simulink model "HFV_Injection_2015a"  (R2016a)
settings: Solver=ode3  SolverMode=SingleTasking  StartTime=0.0  StopTime=5  FixedStep=Simulation_Step  RelTol=1e-3
values from neighbouring files (symbols this model uses):
  Dm = 1e-4    (= 0.0001)    [param.m]
  HF = 400    [param.m]
  Jm = 2e-4    (= 0.0002)    [param.m]
  Ke = 0.002    [param.m]
  ki = wpll^2    (= 15791.3670417)    [param.m]
  kp = 2 * wpll    (= 251.327412287)    [param.m]
  Ld = 0.00019    [aaa.mat]    (also in param.m = 2e-05)
  Lq = 0.00051    [aaa.mat]    (also in param.m = 4e-05)
  omega = 100    [param.m]
  Pn = 4    [param.m]
  Qvalue = 1    [param.m]
  R = 2e-3    (= 0.002)    [param.m]
  tau = 1/Fc/2/pi    (= 0.00795774715459)    [param.m]
  tau_spd = 1/Fspd/2/pi    (= 0.0318309886184)    [param.m]
  Vh = 0.1    [param.m]
  w0 = HF * 2 * pi    (= 2513.27412287)    [param.m]
  wlpf = 20 * 2 * pi    (= 125.663706144)    [param.m]
settings Model: Creator=r720r  LastModifiedBy=Lenovo
settings DebuggingCC: SFUnexpectedBacktrackingDiag=error  SFNoUnconditionalDefaultTransitionDiag=error
settings HardwareCC: ProdWordSize=32  ProdHWDeviceType=Specified
settings SFSimCC: SimUseLocalCustomCode=on
settings RTWCC: RTWUseLocalCustomCode=on
settings GRTTargetCC: TargetLangStandard=C99 (ISO)  GeneratePreprocessorConditionals=Use local settings
settings ConfigComp: CovMetricSettings=dwe  CovHtmlReporting=off  CovSaveCumulativeToWorkspaceVar=off  CovSaveSingleToWorkspaceVar=off  CovModelRefEnable=Off  CovExternalEMLEnable=on

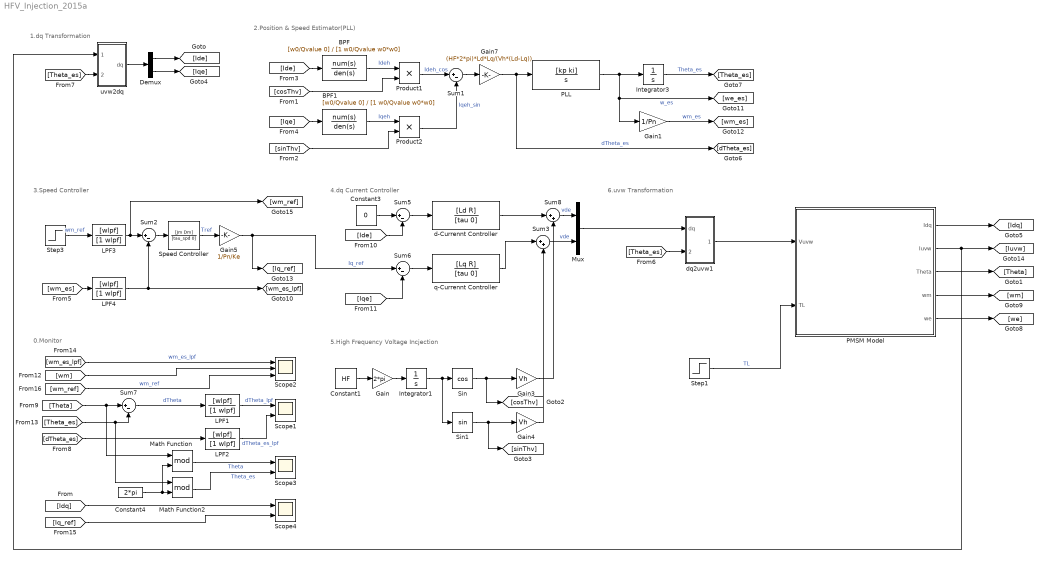
== system HFV_Injection_2015a ==
  note: 0.Monitor
  note: 6.uvw Transformation
  note: 1.dq Transformation
  note: 4.dq Current Controller
  note: 3.Speed Controller
  note: 5.High Frequency Voltage Incjection
  note: 2.Position & Speed Estimator(PLL)
  BPF : TransferFcn  Numerator=[w0/Qvalue 0]  Denominator=[1 w0/Qvalue w0*w0]
  BPF1 : TransferFcn  Numerator=[w0/Qvalue 0]  Denominator=[1 w0/Qvalue w0*w0]
  Constant1 : Constant  Value=HF
  Constant3 : Constant  Value=0
  Constant4 : Constant  Value=2*pi
  Demux : Demux  Outputs=2
  Gain : Gain  Gain=2*pi
  Gain1 : Gain  Gain=1/Pn
  Gain3 : Gain  Gain=Vh
  Gain4 : Gain  Gain=Vh
  Gain5 : Gain  Gain=1/Pn/Ke
  Gain7 : Gain  Gain=(HF*2*pi)*Ld*Lq/(Vh*(Ld-Lq))
  Integrator1 : Integrator
  Integrator3 : Integrator
  LPF{1..4} (4 alike) : TransferFcn  Numerator=[wlpf]  Denominator=[1 wlpf]
  Math Function : Math  Operator=mod  SaturateOnIntegerOverflow=on
  Math Function2 : Math  Operator=mod  SaturateOnIntegerOverflow=on
  Mux : Mux  Inputs=2
  PLL : TransferFcn  Numerator=[kp ki]  Denominator=[1 0]
  PMSM Model : Subsystem
  Product1 : Product
  Product2 : Product
  Scope1 : Scope  NumInputPorts=2
  Scope2 : Scope  NumInputPorts=3
  Scope3 : Scope  NumInputPorts=2
  Scope4 : Scope  NumInputPorts=2
  Sin : Trigonometry  Operator=cos
  Sin1 : Trigonometry
  Speed Controller : TransferFcn  Numerator=[Jm Dm]  Denominator=[tau_spd 0]
  Step1 : Step  Time=3  After=0.01  SampleTime=0
  Step3 : Step  Time=0.2  After=omega/Pn  SampleTime=0
  Sum{1..2,5..7} (5 alike) : Sum  Inputs=|+-
  Sum3 : Sum  Inputs=|++
  Sum8 : Sum  Inputs=|++
  d-Currennt Controller : TransferFcn  Numerator=[Ld R]  Denominator=[tau 0]
  dq2uvw1 : Subsystem
  q-Currennt Controller : TransferFcn  Numerator=[Lq R]  Denominator=[tau 0]
  uvw2dq : Subsystem
  wires:
  Sin/1 -> [cosThv], Gain3/1
  Sin1/1 -> [sinThv], Gain4/1
  Integrator1/1 -> Sin1/1, Sin/1
  Gain/1 -> Integrator1/1
  Constant1/1 -> Gain/1
  [cosThv] -> Product1/2
  BPF/1 -> Product1/1  "Ideh"
  BPF1/1 -> Product2/1  "Iqeh"
  [sinThv] -> Product2/2
  Product1/1 -> Sum1/1  "Ideh_cos"
  Product2/1 -> Sum1/2  "Iqeh_sin"
  Sum1/1 -> Gain7/1
  Gain7/1 -> [dTheta_es], PLL/1  "dTheta_es"
  PLL/1 -> Gain1/1, [we_es], Integrator3/1  "w_es"
  Integrator3/1 -> [Theta_es]  "Theta_es"
  [Ide] -> BPF/1
  [Iqe] -> BPF1/1
  [Theta_es] -> dq2uvw1/2(Theta)
  dq2uvw1/1(uvw) -> PMSM Model/1(Vuvw)
  Sum8/1 -> Mux/1  "vde"
  d-Currennt Controller/1 -> Sum8/1
  Sum3/1 -> Mux/2  "vde"
  q-Currennt Controller/1 -> Sum3/1
  Constant3/1 -> Sum5/1
  Sum5/1 -> d-Currennt Controller/1
  [Ide] -> Sum5/2
  Sum6/1 -> q-Currennt Controller/1
  [Iqe] -> Sum6/2
  [Theta] -> Math Function/1, Sum7/1
  [Theta_es] -> Math Function2/1, Sum7/2
  Gain3/1 -> Sum8/2
  Gain4/1 -> Sum3/2
  Sum7/1 -> LPF1/1  "dTheta"
  LPF1/1 -> Scope1/1  "dTheta_lpf"
  LPF2/1 -> Scope1/2  "dTheta_es_lpf"
  PMSM Model/3(Theta) -> [Theta]
  PMSM Model/5(we) -> [we]
  PMSM Model/4(wm) -> [wm]
  Sum2/1 -> Speed Controller/1
  Gain1/1 -> [wm_es]  "wm_es"
  Speed Controller/1 -> Gain5/1  "Tref"
  Gain5/1 -> Sum6/1, [Iq_ref]  "Iq_ref"
  [wm] -> Scope2/2
  [wm_es] -> LPF4/1
  LPF4/1 -> [wm_es_lpf], Sum2/2
  PMSM Model/2(Iuvw) -> uvw2dq/1(uvw), [Iuvw]
  Mux/1 -> dq2uvw1/1(dq)
  uvw2dq/1(dq) -> Demux/1
  Demux/1 -> [Ide]
  Demux/2 -> [Iqe]
  [Theta_es] -> uvw2dq/2(Theta)
  PMSM Model/1(Idq) -> [Idq]
  [dTheta_es] -> LPF2/1
  Step3/1 -> LPF3/1  "wm_ref"
  LPF3/1 -> [wm_ref], Sum2/1
  Step1/1 -> PMSM Model/2(TL)  "TL"
  Constant4/1 -> Math Function2/2, Math Function/2
  Math Function/1 -> Scope3/1  "Theta"
  Math Function2/1 -> Scope3/2  "Theta_es"
  [Idq] -> Scope4/1
  [Iq_ref] -> Scope4/2
  [wm_es_lpf] -> Scope2/1  "wm_es_lpf"
  [wm_ref] -> Scope2/3  "wm_ref"

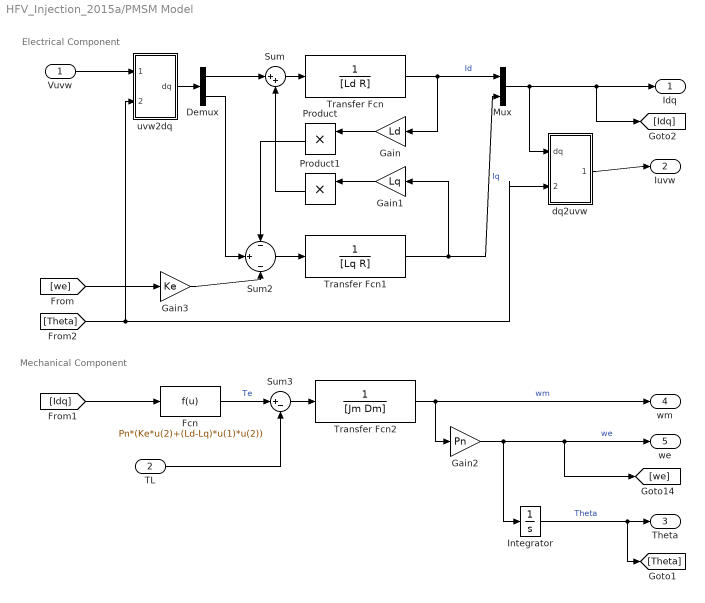
== system HFV_Injection_2015a/PMSM Model ==
  note: Mechanical Component
  note: Electrical Component
  Vuvw : Inport
  TL : Inport  Port=2
  Demux : Demux  Outputs=2
  Fcn : Fcn  Expr=Pn*(Ke*u(2)+(Ld-Lq)*u(1)*u(2))
  Gain : Gain  Gain=Ld
  Gain1 : Gain  Gain=Lq
  Gain2 : Gain  Gain=Pn
  Gain3 : Gain  Gain=Ke
  Integrator : Integrator
  Mux : Mux  Inputs=2
  Product : Product
  Product1 : Product
  Sum : Sum  Inputs=|++
  Sum2 : Sum  Inputs=-|+|-
  Sum3 : Sum  Inputs=|+-
  Transfer Fcn : TransferFcn  Denominator=[Ld R]
  Transfer Fcn1 : TransferFcn  Denominator=[Lq R]
  Transfer Fcn2 : TransferFcn  Denominator=[Jm Dm]
  dq2uvw : Subsystem
  uvw2dq : Subsystem
  Idq : Outport
  Iuvw : Outport  Port=2
  Theta : Outport  Port=3
  wm : Outport  Port=4
  we : Outport  Port=5
  wires:
  Product1/1 -> Sum/2
  Product/1 -> Sum2/1
  Transfer Fcn/1 -> Mux/1, Gain/1  "Id"
  Sum2/1 -> Transfer Fcn1/1
  Gain/1 -> Product/1
  Gain1/1 -> Product1/1
  Sum/1 -> Transfer Fcn/1
  Transfer Fcn1/1 -> Gain1/1, Mux/2  "Iq"
  Vuvw/1 -> uvw2dq/1(uvw)
  Mux/1 -> dq2uvw/1(dq), [Idq], Idq/1
  Fcn/1 -> Sum3/1  "Te"
  Transfer Fcn2/1 -> wm/1, Gain2/1  "wm"
  Gain2/1 -> Integrator/1, we/1, [we]  "we"
  Sum3/1 -> Transfer Fcn2/1
  TL/1 -> Sum3/2
  Gain3/1 -> Sum2/3
  Integrator/1 -> [Theta], Theta/1  "Theta"
  [we] -> Gain3/1
  [Idq] -> Fcn/1
  dq2uvw/1(uvw) -> Iuvw/1
  [Theta] -> dq2uvw/2(Theta), uvw2dq/2(Theta)
  uvw2dq/1(dq) -> Demux/1
  Demux/1 -> Sum/1
  Demux/2 -> Sum2/2

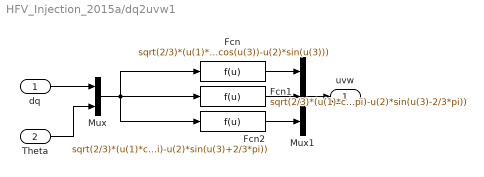
== system HFV_Injection_2015a/dq2uvw1 ==
  dq : Inport
  Theta : Inport  Port=2
  Fcn : Fcn  Expr=sqrt(2/3)*(u(1)*cos(u(3))-u(2)*sin(u(3)))
  Fcn1 : Fcn  Expr=sqrt(2/3)*(u(1)*cos(u(3)-2/3*pi)-u(2)*sin(u(3)-2/3*pi))
  Fcn2 : Fcn  Expr=sqrt(2/3)*(u(1)*cos(u(3)+2/3*pi)-u(2)*sin(u(3)+2/3*pi))
  Mux : Mux  Inputs=2
  Mux1 : Mux  Inputs=3
  uvw : Outport
  wires:
  dq/1 -> Mux/1
  Mux/1 -> Fcn2/1, Fcn/1, Fcn1/1
  Theta/1 -> Mux/2
  Fcn/1 -> Mux1/1
  Fcn1/1 -> Mux1/2
  Fcn2/1 -> Mux1/3
  Mux1/1 -> uvw/1

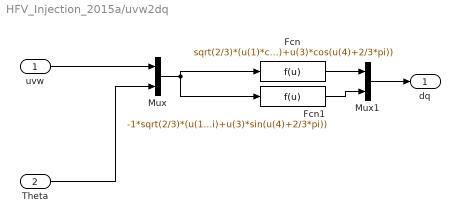
== system HFV_Injection_2015a/uvw2dq ==
  uvw : Inport
  Theta : Inport  Port=2
  Fcn : Fcn  Expr=sqrt(2/3)*(u(1)*cos(u(4))+u(2)*cos(u(4)-2/3*pi)+u(3)*cos(u(4)+2/3*pi))
  Fcn1 : Fcn  Expr=-1*sqrt(2/3)*(u(1)*sin(u(4))+u(2)*sin(u(4)-2/3*pi)+u(3)*sin(u(4)+2/3*pi))
  Mux : Mux  Inputs=2
  Mux1 : Mux  Inputs=2
  dq : Outport
  wires:
  uvw/1 -> Mux/1
  Mux/1 -> Fcn1/1, Fcn/1
  Fcn1/1 -> Mux1/2
  Fcn/1 -> Mux1/1
  Theta/1 -> Mux/2
  Mux1/1 -> dq/1

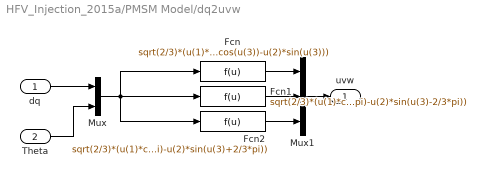
== system HFV_Injection_2015a/PMSM Model/dq2uvw ==
  dq : Inport
  Theta : Inport  Port=2
  Fcn : Fcn  Expr=sqrt(2/3)*(u(1)*cos(u(3))-u(2)*sin(u(3)))
  Fcn1 : Fcn  Expr=sqrt(2/3)*(u(1)*cos(u(3)-2/3*pi)-u(2)*sin(u(3)-2/3*pi))
  Fcn2 : Fcn  Expr=sqrt(2/3)*(u(1)*cos(u(3)+2/3*pi)-u(2)*sin(u(3)+2/3*pi))
  Mux : Mux  Inputs=2
  Mux1 : Mux  Inputs=3
  uvw : Outport
  wires:
  dq/1 -> Mux/1
  Mux/1 -> Fcn2/1, Fcn/1, Fcn1/1
  Theta/1 -> Mux/2
  Fcn/1 -> Mux1/1
  Fcn1/1 -> Mux1/2
  Fcn2/1 -> Mux1/3
  Mux1/1 -> uvw/1

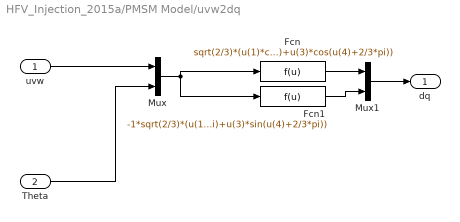
== system HFV_Injection_2015a/PMSM Model/uvw2dq ==
  uvw : Inport
  Theta : Inport  Port=2
  Fcn : Fcn  Expr=sqrt(2/3)*(u(1)*cos(u(4))+u(2)*cos(u(4)-2/3*pi)+u(3)*cos(u(4)+2/3*pi))
  Fcn1 : Fcn  Expr=-1*sqrt(2/3)*(u(1)*sin(u(4))+u(2)*sin(u(4)-2/3*pi)+u(3)*sin(u(4)+2/3*pi))
  Mux : Mux  Inputs=2
  Mux1 : Mux  Inputs=2
  dq : Outport
  wires:
  uvw/1 -> Mux/1
  Mux/1 -> Fcn1/1, Fcn/1
  Fcn1/1 -> Mux1/2
  Fcn/1 -> Mux1/1
  Theta/1 -> Mux/2
  Mux1/1 -> dq/1
